simulink model "timeVaryingPathModel"  (R2017b)
settings: Solver=ode45  StartTime=0.0  StopTime=50  FixedStep=0.001  MaxStep=.01  RelTol=1e-3  AbsTol=1e-7
undefined symbols (not defined in the file or in its folder): sgn
settings Model: Creator=greenoctbass  LastModifiedBy=greenoctbass
settings DataIOCC: SaveFormat=Array  SaveState=on

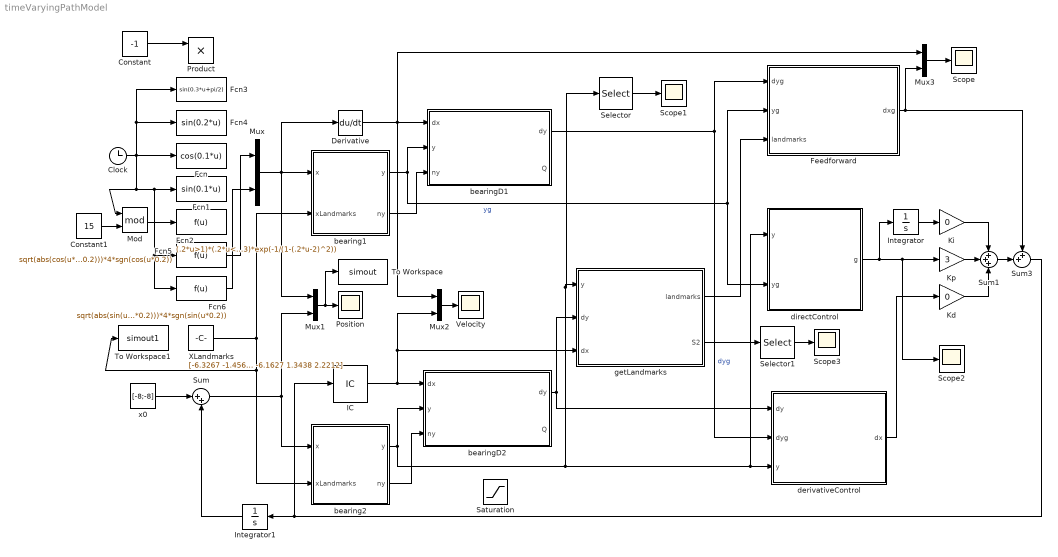
== system timeVaryingPathModel ==
  Clock : Clock
  Constant : Constant  Value=-1
  Constant1 : Constant  Value=15
  Derivative : Derivative
  Fcn : Fcn  Expr=cos(0.1*u)
  Fcn1 : Fcn  Expr=sin(0.1*u)
  Fcn2 : Fcn  Expr=(.2*u>1)*(.2*u<3)*exp(-1/(1-(.2*u-2)^2))
  Fcn3 : Fcn  Expr=sin(0.3*u+pi/2)
  Fcn4 : Fcn  Expr=sin(0.2*u)
  Fcn5 : Fcn  Expr=sqrt(abs(cos(u*0.2)))*4*sgn(cos(u*0.2))
  Fcn6 : Fcn  Expr=sqrt(abs(sin(u*0.2)))*4*sgn(sin(u*0.2))
  Feedforward : MATLAB Function  TreatAsAtomicUnit=on
  IC : InitialCondition  Value=[1;1]
  Integrator : Integrator
  Integrator1 : Integrator
  Kd : Gain  Gain=0
  Ki : Gain  Gain=0
  Kp : Gain  Gain=3
  Mod : Math  Operator=mod  SaturateOnIntegerOverflow=on
  Mux{,1..3} (4 alike) : Mux  Inputs=2
  Position : Scope
  Product : Product
  Saturation : Saturate  UpperLimit=6  LowerLimit=-6
  Scope{,1..3} (4 alike) : Scope
  Selector : Selector  NumberOfDimensions=2  InputPortWidth=3  IndexOptions=Select all,Select all  Indices=[1 3],1  OutputSizes=1,1
  Selector1 : Selector  InputPortWidth=8  IndexOptions=Select all  Indices=[6 7 8]  OutputSizes=1
  Sum : Sum  Inputs=|++
  Sum1 : Sum  Inputs=+++
  Sum3 : Sum  Inputs=++|
  To Workspace : ToWorkspace  VariableName=simout  SaveFormat=Timeseries  SampleTime=-1
  To Workspace1 : ToWorkspace  VariableName=simout1  SaveFormat=Timeseries  SampleTime=-1
  Velocity : Scope
  XLandmarks : Constant  Value=[-6.3267 -1.4564 6.4309 -9.4093 -5.0582 -1.3374; -5.6740 9.4115 -2.6130 -6.1627 1.3438 2.2212]
  bearing1 : MATLAB Function  TreatAsAtomicUnit=on
  bearing2 : MATLAB Function  TreatAsAtomicUnit=on
  bearingD1 : MATLAB Function  TreatAsAtomicUnit=on
  bearingD2 : MATLAB Function  TreatAsAtomicUnit=on
  derivativeControl : MATLAB Function  TreatAsAtomicUnit=on
  directControl : MATLAB Function  TreatAsAtomicUnit=on
  getLandmarks : MATLAB Function  TreatAsAtomicUnit=on
  x0 : Constant  Value=[-8;-8]
  wires:
  XLandmarks/1 -> bearing1/2(xLandmarks), To Workspace1/1, bearing2/2(xLandmarks)
  Mux/1 -> Mux1/1, Derivative/1, bearing1/1(x)
  bearing1/1(y) -> Feedforward/2(yg), directControl/2(yg), bearingD1/2(y)  "yg"
  Derivative/1 -> Mux3/1, bearingD1/1(dx), Mux2/1
  bearing1/2(ny) -> bearingD1/3(ny)
  x0/1 -> Sum/1
  bearing2/2(ny) -> bearingD2/3(ny)
  directControl/1(g) -> Integrator/1, Scope2/1, Kp/1
  Integrator/1 -> Ki/1
  Kp/1 -> Sum1/2
  Ki/1 -> Sum1/1
  Integrator1/1 -> Sum/2
  Mux1/1 -> To Workspace/1, Position/1
  derivativeControl/1(dx) -> Kd/1
  Mux2/1 -> Velocity/1
  bearing2/1(y) -> bearingD2/2(y), Selector/1, getLandmarks/1(y), directControl/1(y), derivativeControl/3(y)
  bearingD1/1(dy) -> derivativeControl/2(dyg), Feedforward/1(dyg)  "dyg"
  getLandmarks/1(landmarks) -> Feedforward/3(landmarks)
  bearingD2/1(dy) -> getLandmarks/2(dy), derivativeControl/1(dy)
  Selector/1 -> Scope1/1
  Mux3/1 -> Scope/1
  Clock/1 -> Mod/1, Fcn5/1, Fcn6/1, Fcn1/1, Fcn/1, Fcn4/1, Fcn3/1
  Constant/1 -> Product/1
  IC/1 -> getLandmarks/3(dx), Mux2/2, bearingD2/1(dx)
  Sum1/1 -> Sum3/2
  getLandmarks/2(S2) -> Selector1/1
  Kd/1 -> Sum1/3
  Selector1/1 -> Scope3/1
  Mod/1 -> Fcn2/1
  Constant1/1 -> Mod/2
  Sum/1 -> Mux1/2, bearing2/1(x)
  Feedforward/1(dxg) -> Sum3/1, Mux3/2
  Sum3/1 -> IC/1, Integrator1/1
  Fcn5/1 -> Mux/1
  Fcn6/1 -> Mux/2

== matlab function timeVaryingPathModel/bearingD1 ==
  data: dx input; dy output; y input; ny input; Q output
%Compute derivative of bearing vectors
%function [dy,Q]=bearingComputeDerivative(dx,y,ny)
%Inputs
%   dx   derivative of robot's location
%   y   current bearings
%   ny  ranges corresponding to the bearings
%Output
%   dy  derivative of Y along v
%   Q   array of matrices such that dY=Q*v
function [dy,Q]=bearingComputeDerivative(dx,y,ny)
flagComputeQ=false;
if nargout>1
    flagComputeQ=true;
end
[d,Ny]=size(y);
dy=zeros(d,Ny);
if flagComputeQ
    Q=zeros(d,d,Ny);
end
I=eye(d);
for iY=1:Ny
    Qi=-inv(ny(iY))*(I-y(:,iY)*y(:,iY)');
    dy(:,iY)=Qi*dx;
    if flagComputeQ
        Q(:,:,iY)=Qi;
    end
end

== matlab function timeVaryingPathModel/bearing1 ==
  data: x input; y output; xLandmarks input; ny output
%Compute bearing information from base point and landmarks
%function [y,ny]=bearingCompute(x,xLandmarks)
%Inputs
%   x           coordinates of base point
%   xLandmarks  coordinates of landmarks
%Outputs
%   y       bearings
%   ny      ranges corresponding to the bearings
%
function [y,ny]=bearingCompute(x,xLandmarks)
Nx=size(x,2);
NxLandmarks=size(xLandmarks,2);
if Nx==1 && NxLandmarks>1
    z=x*ones(1,NxLandmarks);
elseif NxLandmarks==1 && Nx>1
    xLandmarks=xLandmarks*ones(1,Nx);
end
[y,ny]=cnormalize(xLandmarks-z);

== matlab function timeVaryingPathModel/bearing2 ==
  data: x input; y output; xLandmarks input; ny output
%Compute bearing information from base point and landmarks
%function [y,ny]=bearingCompute(x,xLandmarks)
%Inputs
%   x           coordinates of base point
%   xLandmarks  coordinates of landmarks
%Outputs
%   y       bearings
%   ny      ranges corresponding to the bearings
%
function [y,ny]=bearingCompute(x,xLandmarks)
Nx=size(x,2);
NxLandmarks=size(xLandmarks,2);
if Nx==1 && NxLandmarks>1
    z=x*ones(1,NxLandmarks);
elseif NxLandmarks==1 && Nx>1
    xLandmarks=xLandmarks*ones(1,Nx);
end
[y,ny]=cnormalize(xLandmarks-z);

== matlab function timeVaryingPathModel/bearingD2 ==
  data: dx input; dy output; y input; ny input; Q output
%Compute derivative of bearing vectors
%function [dy,Q]=bearingComputeDerivative(dx,y,ny)
%Inputs
%   dx   derivative of robot's location
%   y   current bearings
%   ny  ranges corresponding to the bearings
%Output
%   dy  derivative of Y along v
%   Q   array of matrices such that dY=Q*v
function [dy,Q]=bearingComputeDerivative(dx,y,ny)
flagComputeQ=false;
if nargout>1
    flagComputeQ=true;
end
[d,Ny]=size(y);
dy=zeros(d,Ny);
if flagComputeQ
    Q=zeros(d,d,Ny);
end
I=eye(d);
for iY=1:Ny
    Qi=-inv(ny(iY))*(I-y(:,iY)*y(:,iY)');
    dy(:,iY)=Qi*dx;
    if flagComputeQ
        Q(:,:,iY)=Qi;
    end
end

== matlab function timeVaryingPathModel/directControl ==
  data: y input; g output; yg input
%Compute the velocity control from the bearing potential
%function dx=bearingControlDirect(y,yg,funs)
%Inputs
%   y       Current bearing vectors
%   yg      Goal's bearing vectors
%   funs    Reshaping function for the generalized cost
%
function g=bearingControlDirect(y,yg)
flagPrecondition=false;
funs=bearingCostFunctions('cosine');

%optional parameters
% ivarargin=1;
% while ivarargin<=length(varargin)
%     switch lower(varargin{ivarargin})
%         case 'precondition'
%             flagPrecondition=true;
%         otherwise
%             disp(varargin{ivarargin})
%             error('Argument not valid!')
%     end
%     ivarargin=ivarargin+1;
% end

if ~flagPrecondition
    g=-bearingCostGeneral_gradient_noOptional(y,yg,funs);
else
    g=bearingCostGeneral_gradient(y,yg,funs);
    [~,Hdx]=bearingCostGeneral_gradient_noOptional(y,yg,funs);
    %Hdx=Hdx/det(Hdx);
    g=-Hdx\g;
end

== matlab function timeVaryingPathModel/derivativeControl ==
  data: dy input; dx output; dyg input; y input
function dx = bearingControlDerivative(dy,dyg,y)

[d,Ny]=size(y);
I=eye(d);
Q=zeros(d*Ny,d);
Y=zeros(d*Ny,1);
for iY=1:Ny
    Qi=(I-y(:,iY)*y(:,iY)');
    Y((iY-1)*d+1:d*iY)=Qi*(dy(:,iY)-dyg(:,iY));
    Q(((iY-1)*d+1:d*iY),1:d)=Qi;
end
dx=Q\Y;

== matlab function timeVaryingPathModel/Feedforward ==
  data: dxg output; dyg input; yg input; landmarks input
%Only works for 2d right now - not really, fix it
function dxg    = bearingComputeFeedforward(dyg,yg,landmarks)
[d,Ny]=size(landmarks);
I=eye(d);
xg=zeros(d,1);
dxg=xg;
ny=zeros(Ny,1);
%Q=zeros(d,d*Ny);

%m1=yg(2,1)/yg(1,1);
%m2=yg(2,2)/yg(1,2);
%xgt(1)=(m1*landmarks(1,1)-m2*landmarks(1,2)-landmarks(2,1)+landmarks(2,2))/(m1-m2);
%xgt(2)=m1*(xgt(1)-landmarks(1,1))+landmarks(2,1);
%for iY=1:Ny
%    ny(iY)=norm(landmarks(:,iY)-xg);
%    Qi=-(I-yg(:,iY)*yg(:,iY)')*ny(iY);
%    Q(:,d*(iY-1)+1:d*iY)=Qi;
%end
%z=reshape(dyg,[],1);
%dxg=Q*z;
%test=zeros(2,1);
%test=-dyg*ny;
A=fliplr(yg');
A(:,2)=-A(:,2);
b=sum(A.*landmarks',2);
xg=A\b;
%newyg=yg+dyg;
points=zeros(size(landmarks));
newyg=yg;
for i=1:Ny
    %points(:,i)=xg;
    landmarks(:,i)=landmarks(:,i)-xg;
    points(:,i)=dyg(:,i).*norm(landmarks(:,i));
end
%points=points-landmarks;
A2=fliplr(newyg');
A2(:,2)=-A2(:,2);
b2=sum(A2.*-points',2);
dxg=A2\b2;

== matlab function timeVaryingPathModel/getLandmarks ==
  data: y input; landmarks output; dy input; dx input; S2 output
%Estimate dx and distances to landmarks for dy and Q matrices.
% function [dx,ny]=bearingComputeSVDEstimate(y,dy)
%Inputs
%   y current bearings
%   dy current derivative of bearings (bearingComputeDerivative)
%Outputs
%   dx current estimated derivative of robot's location
%   ny current estimated distances from landmarks
function [landmarks,S2]  = bearingComputeSVDEstimate(y,dy,dx)
[d,Ny]=size(y);
A=zeros(d*Ny,d+Ny);
b=zeros(d+Ny,1);
I=eye(d);
landmarks=zeros(d,Ny);
X=zeros(d,Ny);
for iY=1:Ny
    Qi=(I-y(:,iY)*y(:,iY)');
    A(1+d*(iY-1):d*iY,1:d)=Qi;
    A(1+d*(iY-1):d*iY,iY+d)=dy(:,iY);
end
[~,S,V]=svd(A,'econ');
NS=V(:,Ny+1:end);
alpha=NS(1:d,:)\dx;
v1=NS*alpha;
for i=1:d
    landmarks(i,:)=v1(d+1:end)';
end
landmarks=y.*landmarks;
S2=sum(S,1);
size(S2);
